simulink model "adaptive_lms2"  (Simulink 6.6)
settings: Solver=VariableStepDiscrete  StartTime=0.0  StopTime=15  RelTol=1e-3
StartFcn:
  | tic
StopFcn:
  | toc
libraries: xbsIndex_r4 x26, dspwin32 x2, simulink x1
settings Model: Creator=lcrockett  LastModifiedBy=lcrockett
settings OptimizationCC: InlineParams=on  InlineInvariantSignals=on
settings DebuggingCC: SignalResolutionControl=TryResolveAllWithWarning  MultiTaskDSMMsg=warning  MultiTaskCondExecSysMsg=none  StrictBusMsg=None
settings HardwareCC: TargetHWDeviceType=32-bit Generic  ProdEqTarget=off
settings RTWCC: IncludeERTFirstTime=on

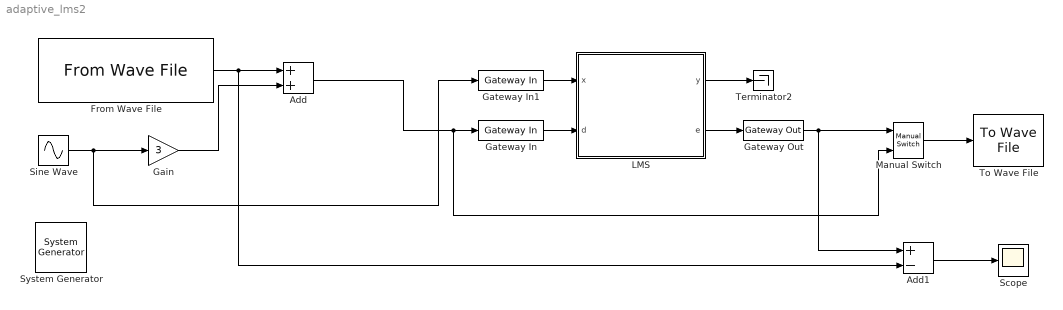
== system adaptive_lms2 ==
  " System Generator" : xbsIndex_r4/ System Generator  Tag=genX  SystemSampleTime=-1  xilinxfamily=Virtex2P  part=xc2vp30  speed=-7  package=ff896  synthesis_tool=XST  clock_wrapper=Clock Enables  directory=./netlist  testbench=off  simulink_period=1/48000  sysclk_period=10  dcm_input_clock_period=100  incr_netlist=off  trim_vbits=Everywhere in SubSystem  dbl_ovrd=According to Block Masks  core_generation=According to Block Masks  run_coregen=off  deprecated_control=off  eval_field=0  block_type=sysgen
      settings: block_version=8.2.01
  Add : Sum  OutScaling=2^-10
  Add1 : Sum  Inputs=+-  OutScaling=2^-10
  From Wave File : dspwin32/From Wave File  FileName=Yabu_sample_48_mono  SamplesPerFrame=1  MinBufSize=1  dType=double  bLoop=off  timesToPlay=1  restartMode=immediately after last sample  firstSampleOutput=off  lastSampleOutput=off
  Gain : Gain  Gain=3
  Gateway In : xbsIndex_r4/Gateway In  arith_type="Signed  (2's comp)"  n_bits=16  bin_pt=13  quantization=Truncate  overflow=Wrap  period=1/48000  dbl_ovrd=off  timing_constraint=None  locs_specified=off  LOCs={}  block_type=gatewayin
      settings: infoedit="Gateway in block.  Converts inputs of type Simulink integer, double and fixed point to  Xilinx fixed point type.<P><P>Hardware notes:  In hardware these blocks become top level input ports."  block_version=8.2.01
  Gateway In1 : xbsIndex_r4/Gateway In  arith_type="Signed  (2's comp)"  n_bits=16  bin_pt=13  quantization=Truncate  overflow=Wrap  period=1/48000  dbl_ovrd=off  timing_constraint=None  locs_specified=off  LOCs={}  block_type=gatewayin
      settings: infoedit="Gateway in block.  Converts inputs of type Simulink integer, double and fixed point to  Xilinx fixed point type.<P><P>Hardware notes:  In hardware these blocks become top level input ports."  block_version=8.2.01
  Gateway Out : xbsIndex_r4/Gateway Out  hdl_port=on  timing_constraint=None  locs_specified=off  LOCs={}  block_type=gatewayout
      settings: infoedit="Gateway out block.  Converts Xilinx fixed point inputs into ouputs of type Simulink integer, double, or fixed point.<P><P>Hardware notes:  In hardware these blocks become top level output ports or are discarded, depending on how they are configured."  block_version=8.2.01
  LMS : Subsystem  mask(LMS Filter){input_bits=16, input_f_bits=13, coeffs=3, coeff_n_bits=20, coeff_f_bits=17, step_size=0.005, step_size_n_bits=14, step_size_f_bits=12, error_n_bits=16, error_f_bits=14, prev_coeffs=3}
      mask prompts: input_bits "Number of bits in input"; input_f_bits "Number of fractional bits in input"; coeffs "Number of coefficients"; coeff_n_bits "Number of bits in coefficients"; coeff_f_bits "Number of fractional bits in coefficients"; step_size "Step size"; step_size_n_bits "Step size number of bits"; step_size_f_bits "Step size number of fractional bits"; error_n_bits "Number of bits in error signal"; error_f_bits "Number of fractional bits in error signal"; prev_coeffs "previous number of coefficients"
      mask help: Adaptive filter using LMS update algorithm
      mask init:
      | sav_gcb=gcb;
      | [bg,fg] = xlcmap('XBlock',0);
      | iPos = get_param(sav_gcb,'Position');
      | iWidth=iPos(3)-iPos(1); iHeight=iPos(4)-iPos(2);
      | iCx=iWidth/2;
      | iCy=iHeight/2;
      | [logoX, logoY] = xlogo(iPos);
      | 
      | % Make sure the entered values for coeffs are positive integers
      | ncoeffs = round(sum(abs(coeffs)));
      | 
      | %set lms_str and use this variable in icon tab to display string in middle of block icon
      | lms_str = sprintf('Adaptive Filter');
      | 
      | % issue an error if the number of coeffs entered is zero
      | if (ncoeffs < 2)
      | 	ncoeffs = prev_coeffs;
      | 	errordlg('Number of Coefficients must be at least 2')
      | end
      | 
      | % issue an error if the number of input fractional bits is greater or equal to the total number of input bits
      | if (input_f_bits >= input_bits)
      | 	errordlg('The number of fractional bits in the input must be less than the number of input bits')
      | end
      | 
      | % issue an error if the number of coefficient fractional bits is greater or equal to the total number of coefficient bits
      | if (coeff_f_bits >= coeff_n_bits)
      | 	errordlg('The number of fractional bits in the coefficients must be less than the number of coefficient bits')
      | end
      | 
      | % issue an error if the number of step size fractional bits is greater or equal to the total number of step size bits
      | if (step_size_f_bits >= step_size_n_bits)
      | 	errordlg('The number of fractional bits in the step size must be less than the number of step size bits')
      | end
      | 
      | % issue an error if the number of error signal fractional bits is greater or equal to the total number of error signal bits
      | if (error_f_bits >= error_n_bits)
      | 	errordlg('The number of fractional bits in the error signal must be less than the number of error signal bits')
      | end
      | 
      | %no change if number of coefficients has not changed
      | if (ncoeffs == prev_coeffs)
      |     return
      | end
      | 
      | %If number of coefficients has changed then delete all connections and blocks (except for first block). 
      | %Then regenerate appropriate number of blocks and reconnect. Finally, reset the parameters for each block.
      | if (ncoeffs ~= prev_coeffs)
      |     
      |     %find instances of mask system LMS Filter in path sav_gcb and assign to handle "update"
      |     update = find_system(sav_gcb, 'lookUnderMasks', 'all', 'FollowLinks','on','masktype', 'LMS Filter');
      |     
      |     %find instances of mask system Update Cell in update and assign to handle "a"
      |     a = find_system(update{1}, 'lookUnderMasks', 'all', 'FollowLinks','on','masktype', 'Update Cell');
      |     
      |     %delete the connections from the final cell to the terminators, y output and error AddSub block
      |     delete_line(update{1}, ['coeff' int2str(length(a)) '/1'], 'Terminator/1');
      |     delete_line(update{1}, ['coeff' int2str(length(a)) '/3'], 'Terminator1/1');
      |     delete_line(update{1}, ['coeff' int2str(length(a)) '/2'], 'y/1');
      |     delete_line(update{1}, ['coeff' int2str(length(a)) '/2'], 'AddSub/2');
      |     
      |     %delete the x, y and z connections from each cell
      |     for i= 2:length(a),
      |         delete_line(update{1}, ['coeff' int2str(i-1) '/1'], ['coeff' int2str(i) '/1']);
      |         delete_line(update{1}, ['coeff' int2str(i-1) '/2'], ['coeff' int2str(i) '/2']);
      |         delete_line(update{1}, ['coeff' int2str(i-1) '/3'], ['coeff' int2str(i) '/3']);
      |     end
      |      
      |     %delete all but first cell
      |     for i=2:length(a),
      |         delete_block([update{1} '/coeff' int2str(i)]);
      |     end
      |     
      |     %regenerate appropriate number of cells by copying the first cell (coeff1) and its parameters.
      |     for i=2:ncoeffs,
      |         add_block([update{1} '/coeff1'], [update{1} '/coeff' int2str(i)], 'position',[250+(i-1)*125, 70, 305+(i-1)*125, 130]);
      |     end
      |     
      |     %set the position of the two terminator blocks and y output port
      |     set_param([update{1} '/' 'Terminator'], 'Position', [250+ncoeffs*125, 72, 266+ncoeffs*125, 88]);
      |     set_param([update{1} '/' 'Terminator1'], 'Position', [250+ncoeffs*125, 112, 266+ncoeffs*125, 128]);
      |     set_param([update{1} '/' 'y'], 'Position', [220+ncoeffs*125, 94, 250+ncoeffs*125, 107]);
      |     
      |     %regenerate x, y and z connections between blocks
      |     for i=2:ncoeffs
      | 		add_line(update{1}, ['coeff' int2str(i-1) '/1'], ['coeff' int2str(i) '/1'], 'autorouting', 'on');
      |         add_line(update{1}, ['coeff' int2str(i-1) '/2'], ['coeff' int2str(i) '/2'], 'autorouting', 'on');
      |         add_line(update{1}, ['coeff' int2str(i-1) '/3'], ['coeff' int2str(i) '/3'], 'autorouting', 'on');
      |     end
      |     
      |     %connect the final cell to the terminator blocks, y output and error AddSub block
      |     add_line(update{1}, ['coeff' int2str(ncoeffs) '/1'], 'Terminator/1', 'autorouting', 'on');
      |     add_line(update{1}, ['coeff' int2str(ncoeffs) '/3'], 'Terminator1/1', 'autorouting', 'on');
      |     add_line(update{1}, ['coeff' int2str(ncoeffs) '/2'], 'y/1', 'autorouting', 'on');
      |     add_line(update{1}, ['coeff' int2str(ncoeffs) '/2'], 'AddSub/2', 'autorouting', 'on');
      |     
      |     %set the width of the FIR adders for each cell except the first one
      |     for i=1:ncoeffs-1,
      | 		set_param([update{1} '/coeff' int2str(i+1)], 'add_n_bits', ['input_bits + coeff_n_bits + 1 + (floor(log2(' int2str(i) ')))']);
      |     end
      | 
      | %     %set the width of the FIR adder in the first cell
      | %     set_param([update{1} '/coeff1'], 'add_n_bits', 'input_bits + coeff_n_bits');
      |     
      |     %if in this "if" statement then need to update the variable prev_coeffs for next execution
      |     set_param(sav_gcb, 'prev_coeffs', int2str(ncoeffs));
      | end
      settings: CopyFcn=set_param(gcb, 'MaskSelfModifiable', 'on', 'LinkStatus', 'none');
      mask Help:
      | This block uses the LMS algorithm to update the filter weights of an FIR filter.
      | 
      | The wordlengths of the internal operators are computed according to the following:
      | 
      | FIR multiplier output width = Input signal width + Coefficient width
      | FIR multiplier fractional output width = Input signal fractional width + Coefficient fractional width
      | 
      | FIR adder chain output width = FIR multiplier output width + 1 + floor(log2(position of adder in chain))
      | FIR adder chain fractional output width = FIR multiplier fractional output width
      | 
      | Feedback multiplier output width = Error signal width + Input signal width
      | Feedback multiplier fractional output width = Error signal fractional width + Input signal fractional width
      mask Display:
      | patch([0 iWidth iWidth 0],[0 0 iHeight iHeight] , bg);
      | patch(logoX,logoY , fg);
      | plot([0 0 iWidth iWidth 0], [0 iHeight iHeight 0 0]);
      | port_label('input',1,'x');
      | port_label('input',2,'d');
      | port_label('output',1,'y');
      | port_label('output',2,'e');
      | disp(lms_str)
  Manual Switch : simulink/Signal Routing/Manual Switch  SystemSampleTime=-1  sw=1  action=0  varsize=off
  Scope : Scope
  Sine Wave : Sin  Amplitude=0.5  Frequency=2*pi*1200  SampleTime=1/48000  VectorParams1D=off
  Terminator2 : Terminator
  To Wave File : dspwin32/To Wave File  filename=audio  sampleWidth=16  MinNumSamples=256
  wires:
  From Wave File/1 -> Add/1, Add1/2
  Sine Wave/1 -> Gain/1, Gateway In1/1
  Add/1 -> Gateway In/1, Manual Switch/2
  Gain/1 -> Add/2
  Gateway In/1 -> LMS/2(d)
  Gateway In1/1 -> LMS/1(x)
  LMS/2(e) -> Gateway Out/1
  LMS/1(y) -> Terminator2/1
  Manual Switch/1 -> To Wave File/1
  Gateway Out/1 -> Manual Switch/1, Add1/1
  Add1/1 -> Scope/1

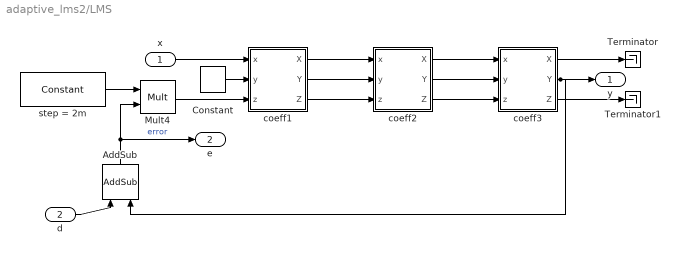
== system adaptive_lms2/LMS ==
  x : Inport
  d : Inport  Port=2
  AddSub : xbsIndex_r4/AddSub  Orientation=up  mode=Subtraction  use_carryin=off  use_carryout=off  en=off  latency=0  precision=User Defined  arith_type="Signed  (2's comp)"  n_bits=error_n_bits  bin_pt=error_f_bits  quantization=Truncate  overflow=Saturate  dbl_ovrd=off  use_behavioral_HDL=on  pipelined=off  use_rpm=on  block_type=addsub
      settings: xl_area=[0, 0, 0, 0, 0, 0, 0]  block_version=VER_STRING_GOES_HERE
  Constant : xbsIndex_r4/Constant  arith_type=Signed (2's comp)  const=0  n_bits=1  bin_pt=0  explicit_period=off  period=1  equ=P=C  opselect=C  inp2=PCIN>>17  opr=+  inp1=P  carry=CIN  dbl_ovrd=off  block_type=constant
      settings: block_version=8.2.01
  Mult4 : xbsIndex_r4/Mult  precision=User Defined  arith_type="Signed  (2's comp)"  n_bits=error_n_bits  bin_pt=error_f_bits  quantization="Round  (unbiased: +/- Inf)"  overflow=Wrap  en=off  latency=0  dbl_ovrd=off  use_behavioral_HDL=off  use_embedded=on  opt=Speed  optimum_pipeline=off  pipeline=off  use_rpm=on  placement_style=Rectangular shape  block_type=mult
      settings: infoedit=Hardware notes: To use the internal pipeline stage of the dedicated multiplier you must select 'Pipeline for maximum performance'.  xl_area=[0, 0, 0, 0, 0, 0, 0]  block_version=VER_STRING_GOES_HERE
  Terminator : Terminator
  Terminator1 : Terminator
  coeff1 : Subsystem  mask(Update Cell){input_bits=input_bits, input_f_bits=input_f_bits, coeff_n_bits=coeff_n_bits, coeff_f_bits=coeff_f_bits, mult_n_bits=input_bits + coeff_n_bits, mult_f_bits=input_f_bits + coeff_f_bits, add_n_bits=input_bits + coeff_n_bits, add_f_bits=input_f_bits + coeff_f_bits, error_n_bits=error_n_bits, error_f_bits=error_f_bits}
      mask prompts: input_bits "Input number of bits"; input_f_bits "Input number of fractional bits"; coeff_n_bits "Number of bits in coefficients"; coeff_f_bits "Number of fractional bits in coefficients"; mult_n_bits "Output width of FIR multipliers"; mult_f_bits "Fractional width of FIR multipliers"; add_n_bits "Output width of FIR adder"; add_f_bits "Fractional width of FIR adder"; error_n_bits "Number of bits in error signal"; error_f_bits "Number of fractional bits in error signal"
      mask init:
      | [bg,fg] = xlcmap('XBlock',0);
      | iPos = get_param(gcb,'Position');
      | iWidth=iPos(3)-iPos(1); iHeight=iPos(4)-iPos(2);
      | iCx=iWidth/2;
      | iCy=iHeight/2;
      | [logoX, logoY] = xlogo(iPos);
      | 
      | set_param(gcb, 'LinkStatus', 'none');
      mask Display:
      | patch([0 iWidth iWidth 0],[0 0 iHeight iHeight] , bg);
      | patch(logoX,logoY , fg);
      | port_label('input',1,'x');
      | port_label('input',2,'y');
      | port_label('input',3,'z');
      | port_label('output',1,'X');
      | port_label('output',2,'Y');
      | port_label('output',3,'Z');
      | plot([0 0 iWidth iWidth 0], [0 iHeight iHeight 0 0]);
  coeff2 : Subsystem  mask(Update Cell){input_bits=input_bits, input_f_bits=input_f_bits, coeff_n_bits=coeff_n_bits, coeff_f_bits=coeff_f_bits, mult_n_bits=input_bits + coeff_n_bits, mult_f_bits=input_f_bits + coeff_f_bits, add_n_bits=input_bits + coeff_n_bits + 1 + (floor(log2(1))), add_f_bits=input_f_bits + coeff_f_bits, error_n_bits=error_n_bits, error_f_bits=error_f_bits}
      mask prompts: input_bits "Input number of bits"; input_f_bits "Input number of fractional bits"; coeff_n_bits "Number of bits in coefficients"; coeff_f_bits "Number of fractional bits in coefficients"; mult_n_bits "Output width of FIR multipliers"; mult_f_bits "Fractional width of FIR multipliers"; add_n_bits "Output width of FIR adder"; add_f_bits "Fractional width of FIR adder"; error_n_bits "Number of bits in error signal"; error_f_bits "Number of fractional bits in error signal"
      mask init: same as adaptive_lms2/LMS/coeff1
      mask Display:
      | patch([0 iWidth iWidth 0],[0 0 iHeight iHeight] , bg);
      | patch(logoX,logoY , fg);
      | port_label('input',1,'x');
      | port_label('input',2,'y');
      | port_label('input',3,'z');
      | port_label('output',1,'X');
      | port_label('output',2,'Y');
      | port_label('output',3,'Z');
      | plot([0 0 iWidth iWidth 0], [0 iHeight iHeight 0 0]);
  coeff3 : Subsystem  mask(Update Cell){input_bits=input_bits, input_f_bits=input_f_bits, coeff_n_bits=coeff_n_bits, coeff_f_bits=coeff_f_bits, mult_n_bits=input_bits + coeff_n_bits, mult_f_bits=input_f_bits + coeff_f_bits, add_n_bits=input_bits + coeff_n_bits + 1 + (floor(log2(2))), add_f_bits=input_f_bits + coeff_f_bits, error_n_bits=error_n_bits, error_f_bits=error_f_bits}
      mask prompts: input_bits "Input number of bits"; input_f_bits "Input number of fractional bits"; coeff_n_bits "Number of bits in coefficients"; coeff_f_bits "Number of fractional bits in coefficients"; mult_n_bits "Output width of FIR multipliers"; mult_f_bits "Fractional width of FIR multipliers"; add_n_bits "Output width of FIR adder"; add_f_bits "Fractional width of FIR adder"; error_n_bits "Number of bits in error signal"; error_f_bits "Number of fractional bits in error signal"
      mask init: same as adaptive_lms2/LMS/coeff1
      mask Display:
      | patch([0 iWidth iWidth 0],[0 0 iHeight iHeight] , bg);
      | patch(logoX,logoY , fg);
      | port_label('input',1,'x');
      | port_label('input',2,'y');
      | port_label('input',3,'z');
      | port_label('output',1,'X');
      | port_label('output',2,'Y');
      | port_label('output',3,'Z');
      | plot([0 0 iWidth iWidth 0], [0 iHeight iHeight 0 0]);
  step = 2m : xbsIndex_r4/Constant  arith_type=Signed (2's comp)  const=step_size  n_bits=step_size_n_bits  bin_pt=step_size_f_bits  explicit_period=off  period=1/10e6  equ=P=C  opselect=C  inp2=PCIN>>17  opr=+  inp1=P  carry=CIN  dbl_ovrd=off  block_type=constant
      settings: block_version=VER_STRING_GOES_HERE
  y : Outport
  e : Outport  Port=2
  wires:
  Constant/1 -> coeff1/2(y)
  d/1 -> AddSub/1
  step = 2m/1 -> Mult4/1
  AddSub/1 -> e/1, Mult4/2  "error"
  x/1 -> coeff1/1(x)
  Mult4/1 -> coeff1/3(z)
  coeff1/1(X) -> coeff2/1(x)
  coeff1/2(Y) -> coeff2/2(y)
  coeff1/3(Z) -> coeff2/3(z)
  coeff2/1(X) -> coeff3/1(x)
  coeff2/2(Y) -> coeff3/2(y)
  coeff2/3(Z) -> coeff3/3(z)
  coeff3/1(X) -> Terminator/1
  coeff3/3(Z) -> Terminator1/1
  coeff3/2(Y) -> y/1, AddSub/2

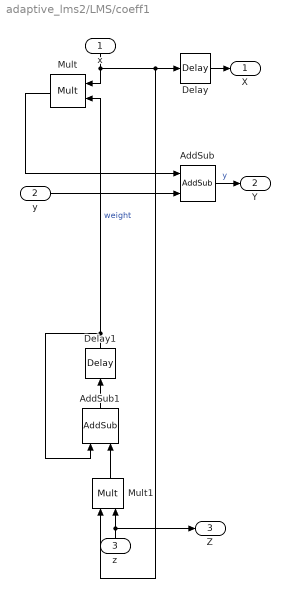
== system adaptive_lms2/LMS/coeff1 ==
  x : Inport  Orientation=down
  y : Inport  Port=2
  z : Inport  Orientation=up  Port=3
  AddSub : xbsIndex_r4/AddSub  mode=Addition  use_carryin=off  use_carryout=off  en=off  latency=0  precision=User Defined  arith_type="Signed  (2's comp)"  n_bits=add_n_bits  bin_pt=add_f_bits  quantization=Truncate  overflow=Wrap  dbl_ovrd=off  use_behavioral_HDL=on  pipelined=off  use_rpm=on  block_type=addsub
      settings: xl_area=[0, 0, 0, 0, 0, 0, 0]  block_version=VER_STRING_GOES_HERE
  AddSub1 : xbsIndex_r4/AddSub  Orientation=up  mode=Addition  use_carryin=off  use_carryout=off  en=off  latency=0  precision=User Defined  arith_type="Signed  (2's comp)"  n_bits=coeff_n_bits  bin_pt=coeff_f_bits  quantization=Truncate  overflow=Saturate  dbl_ovrd=off  use_behavioral_HDL=on  pipelined=off  use_rpm=on  block_type=addsub
      settings: xl_area=[0, 0, 0, 0, 0, 0, 0]  block_version=VER_STRING_GOES_HERE
  Delay : xbsIndex_r4/Delay  en=off  latency=1  dbl_ovrd=off  reg_retiming=on  block_type=delay
      settings: infoedit=Hardware notes: A delay line is a chain, each link of which is an SRL16 followed by a flip-flop. If register retiming is enabled, the delay line is a chain of flip-flops.  xl_area=[0, 0, 0, 0, 0, 0, 0]  block_version=VER_STRING_GOES_HERE
  Delay1 : xbsIndex_r4/Delay  Orientation=up  en=off  latency=1  dbl_ovrd=off  reg_retiming=on  block_type=delay
      settings: infoedit=Hardware notes: A delay line is a chain, each link of which is an SRL16 followed by a flip-flop. If register retiming is enabled, the delay line is a chain of flip-flops.  xl_area=[0, 0, 0, 0, 0, 0, 0]  block_version=VER_STRING_GOES_HERE
  Mult : xbsIndex_r4/Mult  Orientation=left  precision=User Defined  arith_type="Signed  (2's comp)"  n_bits=mult_n_bits  bin_pt=mult_f_bits  quantization=Truncate  overflow=Wrap  en=off  latency=0  dbl_ovrd=off  use_behavioral_HDL=off  use_embedded=on  opt=Speed  optimum_pipeline=off  pipeline=off  use_rpm=on  placement_style=Rectangular shape  block_type=mult
      settings: infoedit=Hardware notes: To use the internal pipeline stage of the dedicated multiplier you must select 'Pipeline for maximum performance'.  xl_area=[0, 0, 0, 0, 0, 0, 0]  block_version=VER_STRING_GOES_HERE
  Mult1 : xbsIndex_r4/Mult  Orientation=up  precision=User Defined  arith_type="Signed  (2's comp)"  n_bits=error_n_bits + input_bits  bin_pt=error_f_bits + input_f_bits  quantization=Truncate  overflow=Wrap  en=off  latency=0  dbl_ovrd=off  use_behavioral_HDL=off  use_embedded=on  opt=Speed  optimum_pipeline=off  pipeline=off  use_rpm=on  placement_style=Rectangular shape  block_type=mult
      settings: infoedit=Hardware notes: To use the internal pipeline stage of the dedicated multiplier you must select 'Pipeline for maximum performance'.  xl_area=[0, 0, 0, 0, 0, 0, 0]  block_version=VER_STRING_GOES_HERE
  X : Outport
  Y : Outport  Port=2
  Z : Outport  Port=3
  wires:
  AddSub1/1 -> Delay1/1
  Delay1/1 -> AddSub1/1, Mult/2  "weight"
  Mult1/1 -> AddSub1/2
  Mult/1 -> AddSub/1
  x/1 -> Mult/1, Mult1/1, Delay/1
  y/1 -> AddSub/2
  AddSub/1 -> Y/1  "y"
  z/1 -> Mult1/2, Z/1
  Delay/1 -> X/1

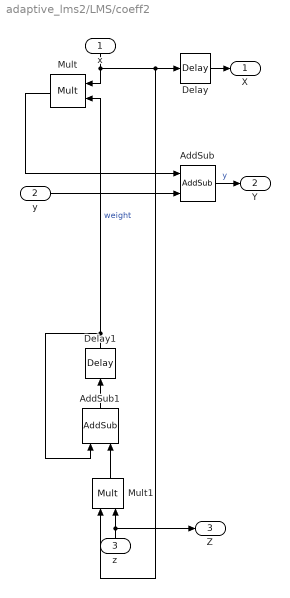
== system adaptive_lms2/LMS/coeff2 ==
  x : Inport  Orientation=down
  y : Inport  Port=2
  z : Inport  Orientation=up  Port=3
  AddSub : xbsIndex_r4/AddSub  mode=Addition  use_carryin=off  use_carryout=off  en=off  latency=0  precision=User Defined  arith_type="Signed  (2's comp)"  n_bits=add_n_bits  bin_pt=add_f_bits  quantization=Truncate  overflow=Wrap  dbl_ovrd=off  use_behavioral_HDL=on  pipelined=off  use_rpm=on  block_type=addsub
      settings: xl_area=[0, 0, 0, 0, 0, 0, 0]  block_version=VER_STRING_GOES_HERE
  AddSub1 : xbsIndex_r4/AddSub  Orientation=up  mode=Addition  use_carryin=off  use_carryout=off  en=off  latency=0  precision=User Defined  arith_type="Signed  (2's comp)"  n_bits=coeff_n_bits  bin_pt=coeff_f_bits  quantization=Truncate  overflow=Saturate  dbl_ovrd=off  use_behavioral_HDL=on  pipelined=off  use_rpm=on  block_type=addsub
      settings: xl_area=[0, 0, 0, 0, 0, 0, 0]  block_version=VER_STRING_GOES_HERE
  Delay : xbsIndex_r4/Delay  en=off  latency=1  dbl_ovrd=off  reg_retiming=on  block_type=delay
      settings: infoedit=Hardware notes: A delay line is a chain, each link of which is an SRL16 followed by a flip-flop. If register retiming is enabled, the delay line is a chain of flip-flops.  xl_area=[0, 0, 0, 0, 0, 0, 0]  block_version=VER_STRING_GOES_HERE
  Delay1 : xbsIndex_r4/Delay  Orientation=up  en=off  latency=1  dbl_ovrd=off  reg_retiming=on  block_type=delay
      settings: infoedit=Hardware notes: A delay line is a chain, each link of which is an SRL16 followed by a flip-flop. If register retiming is enabled, the delay line is a chain of flip-flops.  xl_area=[0, 0, 0, 0, 0, 0, 0]  block_version=VER_STRING_GOES_HERE
  Mult : xbsIndex_r4/Mult  Orientation=left  precision=User Defined  arith_type="Signed  (2's comp)"  n_bits=mult_n_bits  bin_pt=mult_f_bits  quantization=Truncate  overflow=Wrap  en=off  latency=0  dbl_ovrd=off  use_behavioral_HDL=off  use_embedded=on  opt=Speed  optimum_pipeline=off  pipeline=off  use_rpm=on  placement_style=Rectangular shape  block_type=mult
      settings: infoedit=Hardware notes: To use the internal pipeline stage of the dedicated multiplier you must select 'Pipeline for maximum performance'.  xl_area=[0, 0, 0, 0, 0, 0, 0]  block_version=VER_STRING_GOES_HERE
  Mult1 : xbsIndex_r4/Mult  Orientation=up  precision=User Defined  arith_type="Signed  (2's comp)"  n_bits=error_n_bits + input_bits  bin_pt=error_f_bits + input_f_bits  quantization=Truncate  overflow=Wrap  en=off  latency=0  dbl_ovrd=off  use_behavioral_HDL=off  use_embedded=on  opt=Speed  optimum_pipeline=off  pipeline=off  use_rpm=on  placement_style=Rectangular shape  block_type=mult
      settings: infoedit=Hardware notes: To use the internal pipeline stage of the dedicated multiplier you must select 'Pipeline for maximum performance'.  xl_area=[0, 0, 0, 0, 0, 0, 0]  block_version=VER_STRING_GOES_HERE
  X : Outport
  Y : Outport  Port=2
  Z : Outport  Port=3
  wires:
  Delay/1 -> X/1
  z/1 -> Z/1, Mult1/2
  AddSub/1 -> Y/1  "y"
  y/1 -> AddSub/2
  x/1 -> Delay/1, Mult1/1, Mult/1
  Mult/1 -> AddSub/1
  Mult1/1 -> AddSub1/2
  Delay1/1 -> Mult/2, AddSub1/1  "weight"
  AddSub1/1 -> Delay1/1

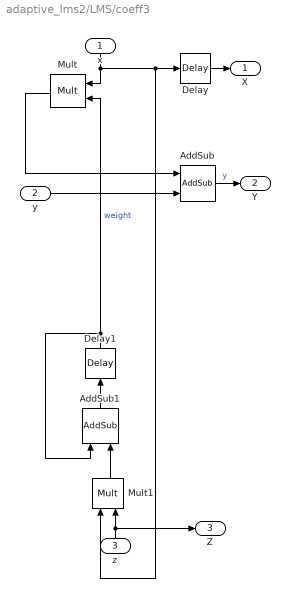
== system adaptive_lms2/LMS/coeff3 ==
  x : Inport  Orientation=down
  y : Inport  Port=2
  z : Inport  Orientation=up  Port=3
  AddSub : xbsIndex_r4/AddSub  mode=Addition  use_carryin=off  use_carryout=off  en=off  latency=0  precision=User Defined  arith_type="Signed  (2's comp)"  n_bits=add_n_bits  bin_pt=add_f_bits  quantization=Truncate  overflow=Wrap  dbl_ovrd=off  use_behavioral_HDL=on  pipelined=off  use_rpm=on  block_type=addsub
      settings: xl_area=[0, 0, 0, 0, 0, 0, 0]  block_version=VER_STRING_GOES_HERE
  AddSub1 : xbsIndex_r4/AddSub  Orientation=up  mode=Addition  use_carryin=off  use_carryout=off  en=off  latency=0  precision=User Defined  arith_type="Signed  (2's comp)"  n_bits=coeff_n_bits  bin_pt=coeff_f_bits  quantization=Truncate  overflow=Saturate  dbl_ovrd=off  use_behavioral_HDL=on  pipelined=off  use_rpm=on  block_type=addsub
      settings: xl_area=[0, 0, 0, 0, 0, 0, 0]  block_version=VER_STRING_GOES_HERE
  Delay : xbsIndex_r4/Delay  en=off  latency=1  dbl_ovrd=off  reg_retiming=on  block_type=delay
      settings: infoedit=Hardware notes: A delay line is a chain, each link of which is an SRL16 followed by a flip-flop. If register retiming is enabled, the delay line is a chain of flip-flops.  xl_area=[0, 0, 0, 0, 0, 0, 0]  block_version=VER_STRING_GOES_HERE
  Delay1 : xbsIndex_r4/Delay  Orientation=up  en=off  latency=1  dbl_ovrd=off  reg_retiming=on  block_type=delay
      settings: infoedit=Hardware notes: A delay line is a chain, each link of which is an SRL16 followed by a flip-flop. If register retiming is enabled, the delay line is a chain of flip-flops.  xl_area=[0, 0, 0, 0, 0, 0, 0]  block_version=VER_STRING_GOES_HERE
  Mult : xbsIndex_r4/Mult  Orientation=left  precision=User Defined  arith_type="Signed  (2's comp)"  n_bits=mult_n_bits  bin_pt=mult_f_bits  quantization=Truncate  overflow=Wrap  en=off  latency=0  dbl_ovrd=off  use_behavioral_HDL=off  use_embedded=on  opt=Speed  optimum_pipeline=off  pipeline=off  use_rpm=on  placement_style=Rectangular shape  block_type=mult
      settings: infoedit=Hardware notes: To use the internal pipeline stage of the dedicated multiplier you must select 'Pipeline for maximum performance'.  xl_area=[0, 0, 0, 0, 0, 0, 0]  block_version=VER_STRING_GOES_HERE
  Mult1 : xbsIndex_r4/Mult  Orientation=up  precision=User Defined  arith_type="Signed  (2's comp)"  n_bits=error_n_bits + input_bits  bin_pt=error_f_bits + input_f_bits  quantization=Truncate  overflow=Wrap  en=off  latency=0  dbl_ovrd=off  use_behavioral_HDL=off  use_embedded=on  opt=Speed  optimum_pipeline=off  pipeline=off  use_rpm=on  placement_style=Rectangular shape  block_type=mult
      settings: infoedit=Hardware notes: To use the internal pipeline stage of the dedicated multiplier you must select 'Pipeline for maximum performance'.  xl_area=[0, 0, 0, 0, 0, 0, 0]  block_version=VER_STRING_GOES_HERE
  X : Outport
  Y : Outport  Port=2
  Z : Outport  Port=3
  wires:
  Delay/1 -> X/1
  z/1 -> Z/1, Mult1/2
  AddSub/1 -> Y/1  "y"
  y/1 -> AddSub/2
  x/1 -> Delay/1, Mult1/1, Mult/1
  Mult/1 -> AddSub/1
  Mult1/1 -> AddSub1/2
  Delay1/1 -> Mult/2, AddSub1/1  "weight"
  AddSub1/1 -> Delay1/1
